simulink model "test5"  (R2018b)
settings: Solver=VariableStepAuto  StartTime=0.0  StopTime=5  RelTol=1e-3
libraries: simulink x4
settings Model: Creator=12732  LastModifiedBy=12732

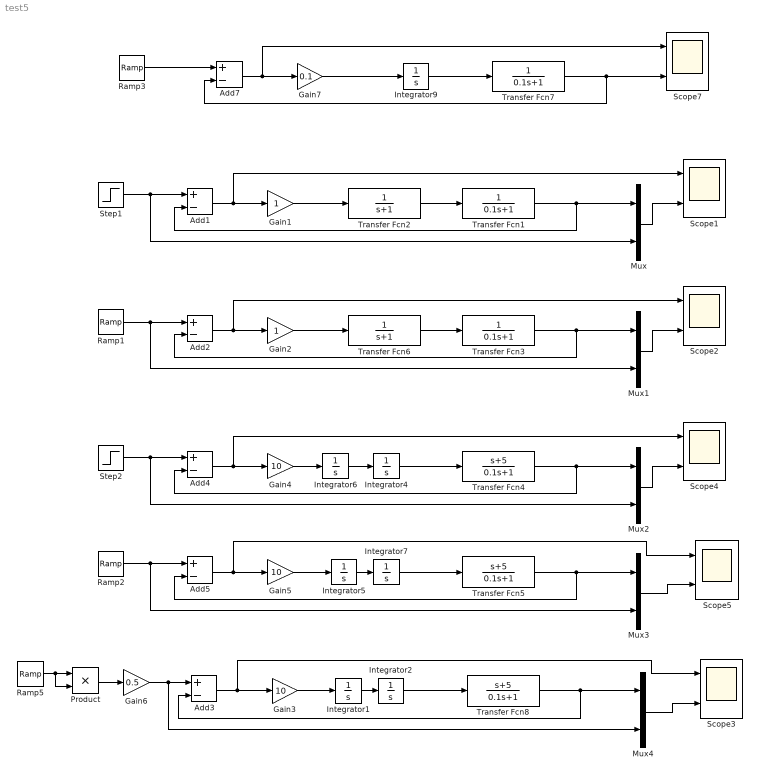
== system test5 ==
  Add{1..5,7} (6 alike) : Sum  Inputs=+-
  Gain1 : Gain
  Gain2 : Gain
  Gain3 : Gain  Gain=10
  Gain4 : Gain  Gain=10
  Gain5 : Gain  Gain=10
  Gain6 : Gain  Gain=0.5
  Gain7 : Gain  Gain=0.1
  Integrator{1..2,4..7,9} (7 alike) : Integrator
  Mux{,1..4} (5 alike) : Mux  Inputs=2
  Product : Product
  Ramp{1..3,5} (4 alike) : simulink/Sources/Ramp  slope=1  start=0  InitialOutput=0
  Scope{1..5,7} (6 alike) : Scope  NumInputPorts=2
  Step1 : Step  SampleTime=0
  Step2 : Step  SampleTime=0
  Transfer Fcn1 : TransferFcn  Denominator=[0.1 1]
  Transfer Fcn2 : TransferFcn  Denominator=[1 1]
  Transfer Fcn3 : TransferFcn  Denominator=[0.1 1]
  Transfer Fcn4 : TransferFcn  Numerator=[1 5]  Denominator=[0.1 1]
  Transfer Fcn5 : TransferFcn  Numerator=[1 5]  Denominator=[0.1 1]
  Transfer Fcn6 : TransferFcn  Denominator=[1 1]
  Transfer Fcn7 : TransferFcn  Denominator=[0.1 1]
  Transfer Fcn8 : TransferFcn  Numerator=[1 5]  Denominator=[0.1 1]
  wires:
  Step1/1 -> Mux/2, Add1/1
  Transfer Fcn1/1 -> Add1/2, Mux/1
  Transfer Fcn2/1 -> Transfer Fcn1/1
  Gain1/1 -> Transfer Fcn2/1
  Add1/1 -> Gain1/1, Scope1/1
  Mux/1 -> Scope1/2
  Ramp2/1 -> Mux3/2, Add5/1
  Transfer Fcn5/1 -> Add5/2, Mux3/1
  Integrator5/1 -> Integrator7/1
  Gain5/1 -> Integrator5/1
  Add5/1 -> Gain5/1, Scope5/1
  Mux3/1 -> Scope5/2
  Mux2/1 -> Scope4/2
  Add4/1 -> Scope4/1, Gain4/1
  Gain4/1 -> Integrator6/1
  Integrator4/1 -> Transfer Fcn4/1
  Transfer Fcn4/1 -> Mux2/1, Add4/2
  Step2/1 -> Add4/1, Mux2/2
  Integrator6/1 -> Integrator4/1
  Integrator7/1 -> Transfer Fcn5/1
  Add7/1 -> Scope7/1, Gain7/1
  Gain7/1 -> Integrator9/1
  Integrator9/1 -> Transfer Fcn7/1
  Transfer Fcn7/1 -> Add7/2, Scope7/2
  Ramp3/1 -> Add7/1
  Mux1/1 -> Scope2/2
  Add2/1 -> Scope2/1, Gain2/1
  Gain2/1 -> Transfer Fcn6/1
  Transfer Fcn6/1 -> Transfer Fcn3/1
  Transfer Fcn3/1 -> Mux1/1, Add2/2
  Ramp1/1 -> Add2/1, Mux1/2
  Integrator2/1 -> Transfer Fcn8/1
  Mux4/1 -> Scope3/2
  Add3/1 -> Scope3/1, Gain3/1
  Gain3/1 -> Integrator1/1
  Integrator1/1 -> Integrator2/1
  Transfer Fcn8/1 -> Mux4/1, Add3/2
  Ramp5/1 -> Product/2, Product/1
  Product/1 -> Gain6/1
  Gain6/1 -> Mux4/2, Add3/1
